simulink model "exampleModel"  (R2017b)
settings: Solver=VariableStepAuto  StartTime=0.0  StopTime=10e-6  RelTol=1e-3
PreLoadFcn:
  | setup
values from neighbouring files (symbols this model uses):
  axiClk = 156.25e6    (= 156250000)    [setup.m]    (also in setup_exampleModel_bus_axi_simulink.m; setup_exampleModel_bus_axi_simulink_lcls2.m; setup_lcls2_pcav.m)
  cav1p1_addr = 204    [setup_exampleModel_bus_axi_simulink.m]    (also in setup_exampleModel_bus_axi_simulink_lcls2.m; setup_lcls2_pcav.m; sysgen_signal.m)
  cav1p2_addr = cav1p1_addr * 2    (= 408)    [setup_exampleModel_bus_axi_simulink.m]    (also in setup_exampleModel_bus_axi_simulink_lcls2.m; setup_lcls2_pcav.m; sysgen_signal.m)
  cav2p1_addr = cav1p1_addr * 3    (= 612)    [setup_exampleModel_bus_axi_simulink.m]    (also in setup_exampleModel_bus_axi_simulink_lcls2.m; setup_lcls2_pcav.m; sysgen_signal.m)
  cav2p2_addr = cav1p1_addr * 4    (= 816)    [setup_exampleModel_bus_axi_simulink.m]    (also in setup_exampleModel_bus_axi_simulink_lcls2.m; setup_lcls2_pcav.m; sysgen_signal.m)
  Fadc = Fs/interleavedChannels    (= 29750000)    [setup.m]    (also in setup_exampleModel_bus_axi_simulink.m = 357000000; setup_exampleModel_bus_axi_simulink_lcls2.m = 351000000; setup_lcls2_pcav.m = 357000000)
  Fproc = 204e6    (= 204000000)    [setup_exampleModel_bus_axi_simulink.m]    (also in setup_exampleModel_bus_axi_simulink_lcls2.m = 200571400; setup_lcls2_pcav.m)
  Tadc = 1/fadc    (= 2.80112044818e-09)    [cavity_signal.m]    (also in setup_exampleModel_bus_axi_simulink.m; setup_exampleModel_bus_axi_simulink_lcls2.m = 2.849002849e-09; setup_lcls2_pcav.m; setup_pcav_simulink.m)
undefined symbols (not defined in the file or in its folder): AXI4, Lite
libraries: xbsIndex_r4 x248, llrf_lib x10, simulink x3
(part 2 of 3)

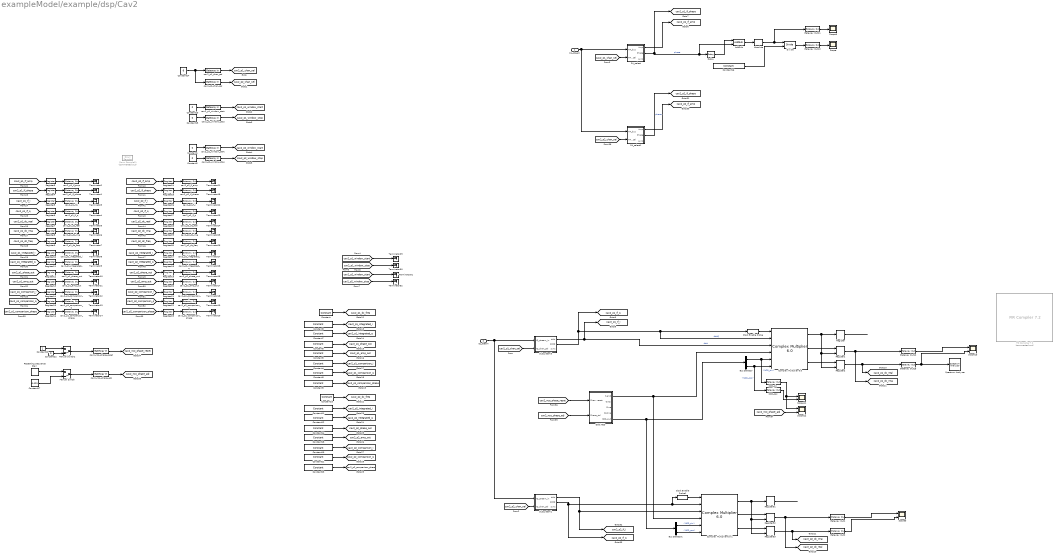
== system exampleModel/example/dsp/Cav2 ==
  PA_stream : Inport
  IQ_stream : Inport  Port=2
  Absolute : xbsIndex_r4/Absolute  precision=Full  arith_type=Unsigned  n_bits=16  bin_pt=14  quantization=Truncate  overflow=Wrap  en=off  latency=1  dbl_ovrd=off  block_type=abs
  AddSub : xbsIndex_r4/AddSub  mode=Subtraction  use_carryin=off  use_carryout=off  en=off  latency=1  precision=Full  arith_type=Unsigned  n_bits=16  bin_pt=14  quantization=Truncate  overflow=Wrap  use_behavioral_HDL=off  hw_selection=Fabric  pipelined=off  dbl_ovrd=off  block_type=addsub
  Bus Selector : BusSelector  OutputSignals=NCO_sin,NCO_cos
  Bus Selector1 : BusSelector  OutputSignals=NCO_sin,NCO_cos
  Clock Enable Probe : xbsIndex_r4/Clock Enable Probe  inherit_constraints=on  block_type=ceprobe
      settings: infoedit="Clock enable extractor.  Produces a Boolean output that mirrors the hardware clock enable associated with the input sample rate.<br><br>Hardware notes: in hardware this block costs nothing."
  Clock Enable Probe1 : xbsIndex_r4/Clock Enable Probe  inherit_constraints=on  block_type=ceprobe
      settings: infoedit="Clock enable extractor.  Produces a Boolean output that mirrors the hardware clock enable associated with the input sample rate.<br><br>Hardware notes: in hardware this block costs nothing."
  "Complex Multiplier 6.0 " : xbsIndex_r4/Complex Multiplier 6.0   hasatlast=off  hasatuser=off  atuserwidth=1  hasbtlast=off  hasbtuser=off  btuserwidth=1  multtype=Use_Mults  optimizegoal=Resources  flowcontrol=NonBlocking  outputwidth=33  roundmode=Truncate  hasctrltlast=off  hasctrltuser=off  ctrltuserwidth=1  outtlastbehv=Null  latencyconfig=Automatic  minimumlatency=15  aclken=off  aresetn=off  trim_axipin_name=on  simulation_type=hybrid_sim  simulation_model=sysgen:cmpy_v6_0  data_path_portlist={ 's_axis_a_tdata_real', 's_axis_a_tdata_imag', 's_axis_b_tdata_real', 's_axis_b_tdata_imag', 's_axis_ctrl_tdata_rounding_bit', 'm_axis_dout_tdata_real', 'm_axis_dout_tdata_imag' }  aportwidth=63  bportwidth=63  ip_name=Complex Multiplier  ip_version=6.0  dsptool_ready=true  ipcore_usecache=true  ipcore_useipmodelcache=true  ipcore_verbose=false  ipcore_latency_parameter='minimumlatency'  wrapper_available=true  port_translation_map={ 'aclken' => 'en', 'aresetn' => 'rst'}  block_type=cmpy_v6_0
  Complex Multiplier 6.0 1 : xbsIndex_r4/Complex Multiplier 6.0   hasatlast=off  hasatuser=off  atuserwidth=1  hasbtlast=off  hasbtuser=off  btuserwidth=1  multtype=Use_Mults  optimizegoal=Resources  flowcontrol=NonBlocking  outputwidth=33  roundmode=Truncate  hasctrltlast=off  hasctrltuser=off  ctrltuserwidth=1  outtlastbehv=Null  latencyconfig=Automatic  minimumlatency=15  aclken=off  aresetn=off  trim_axipin_name=on  simulation_type=hybrid_sim  simulation_model=sysgen:cmpy_v6_0  data_path_portlist={ 's_axis_a_tdata_real', 's_axis_a_tdata_imag', 's_axis_b_tdata_real', 's_axis_b_tdata_imag', 's_axis_ctrl_tdata_rounding_bit', 'm_axis_dout_tdata_real', 'm_axis_dout_tdata_imag' }  aportwidth=63  bportwidth=63  ip_name=Complex Multiplier  ip_version=6.0  dsptool_ready=true  ipcore_usecache=true  ipcore_useipmodelcache=true  ipcore_verbose=false  ipcore_latency_parameter='minimumlatency'  wrapper_available=true  port_translation_map={ 'aclken' => 'en', 'aresetn' => 'rst'}  block_type=cmpy_v6_0
  Constant : xbsIndex_r4/Constant  const=1.0  gui_display_data_type=Fixed-point  arith_type=Signed (2's comp)  n_bits=26  bin_pt=0  preci_type=Single  exp_width=8  frac_width=24  explicit_period=on  period=1/Fproc  equ=P=C  opselect=C  inp2=PCIN>>17  opr=+  inp1=P  carry=CIN  dbl_ovrd=off  block_type=constant
  Constant{1..2,13,15,22} (5 alike) : Constant  Value=0
  Constant10 : xbsIndex_r4/Constant  const=1.0  gui_display_data_type=Fixed-point  arith_type=Signed (2's comp)  n_bits=26  bin_pt=0  preci_type=Single  exp_width=8  frac_width=24  explicit_period=on  period=1/Fproc  equ=P=C  opselect=C  inp2=PCIN>>17  opr=+  inp1=P  carry=CIN  dbl_ovrd=off  block_type=constant
  Constant{3..9,11..12,14,18..19,21,23} (14 alike) : xbsIndex_r4/Constant  const=1.0  gui_display_data_type=Fixed-point  arith_type=Signed (2's comp)  n_bits=18  bin_pt=17  preci_type=Single  exp_width=8  frac_width=24  explicit_period=on  period=1/Fproc  equ=P=C  opselect=C  inp2=PCIN>>17  opr=+  inp1=P  carry=CIN  dbl_ovrd=off  block_type=constant
  Constant16 : xbsIndex_r4/Constant  const=1/(17e6)  gui_display_data_type=Fixed-point  arith_type=Signed (2's comp)  n_bits=32  bin_pt=31  preci_type=Single  exp_width=8  frac_width=24  explicit_period=on  period=1  equ=P=C  opselect=C  inp2=PCIN>>17  opr=+  inp1=P  carry=CIN  dbl_ovrd=off  block_type=constant
  Constant17 : Constant  Value=0.023
  Constant20 : Constant
  Constant24 : Constant  Value=6
  DDC NCO : Subsystem
  Delay : xbsIndex_r4/Delay  rst=off  infoeditControl=Selection of Reset will increase slice count due to use of real FFs and instead of SRLs  en=off  latency=1  reg_retiming=off  dbl_ovrd=off  block_type=delay
  Divide : xbsIndex_r4/Divide  flow_control=NonBlocking  axi_optimize_goal=Resources  algorithm_type=Radix2  infoedit1=Specify output fraction-width for Fixed-point division.  fractional_width=12  infoedit2=Specify latency for Floating-point division.  latency=1  rate=1  has_a_tlast=off  has_a_tuser=off  has_b_tlast=off  has_b_tuser=off  en=off  has_result_tready=off  result_tlast_behv=Pass_A_TLAST  has_underflow=off  has_overflow=off  has_invalid_op=off  has_divide_by_zero=off  fpo_op_type=mergeddivide  block_type=divide
      settings: infoedit=Blocking: Wait for data on all inputs, allow back-pressure.<br>NonBlocking: operate every cycle in which all inputs are valid, no back-pressure.
  Down Sample11 : xbsIndex_r4/Down Sample  Commented=on  sample_ratio=8  sample_phase="Last Value of Frame  (most efficient)"  en=off  rst=off  latency=1  dbl_ovrd=off  block_type=dsamp
  "FIR Compiler 7.2 " : xbsIndex_r4/FIR Compiler 7.2   Commented=on  coefficientvector=[6,0,-4,-3,5,6,-6,-13,7,44,64,44,7,-13,-6,6,5,-3,-4,0,6]  coefficient_sets=1  coefficient_reload=off  filter_type=Single_Rate  rate_change_type=Integer  interpolation_rate=1  decimation_rate=1  zero_pack_factor=1  channel_sequence=Basic  number_channels=1  pattern_list='P4-0,P4-1,P4-2,P4-3,P4-4'  number_paths=1  ratespecification=Maximum_Possible  sampleperiod=1  hardwareoversamplingrate=1  coefficient_sign=Signed  quantization=Integer_Coefficients  coefficient_width=16  bestprecision=on  coefficient_fractional_bits=0  coefficient_structure=Inferred  output_rounding_mode=Full_Precision  output_width=24  filter_architecture=Systolic_Multiply_Accumulate  optimization_goal=Area  optimization_list='None'  data_buffer_type=Automatic  coefficient_buffer_type=Automatic  input_buffer_type=Automatic  output_buffer_type=Automatic  preference_for_other_storage=Automatic  multi_column_support=Automatic  columnconfig='1'  inter_column_pipe_length=4  data_has_tlast=Not_Required  m_data_has_tready=off  s_data_has_fifo=off  s_data_has_tuser=Not_Required  m_data_has_tuser=Not_Required  s_config_sync_mode=On_Vector  s_config_method=Single  num_reload_slots=1  has_aclken=off  has_aresetn=off  infoeditControl=ARESETn must be asserted for a minimum of 2 cycles  reset_data_vector=on  trim_axipin_name=on  simulation_type=hybrid_sim  simulation_model=sysgen:xfirv7_2_cmodel  data_path_portlist={ 's_axis_data_tdata', 'm_axis_data_tdata' }  passband_min=0.0  passband_max=0.5  stopband_min=0.5  stopband_max=1.0  filter_selection=1  gui_behaviour=Sysgen_GUI  data_sign=Signed  data_width=16  data_fractional_bits=0  data_tuser_width=1  wrapper_available=true  ip_wrap_arbitrary_binary_point=true  ip_name=FIR Compiler  ip_version=7.2  dsptool_ready=true  ipcore_usecache=true  ipcore_useipmodelcache=true  port_translation_map={ 'aclken' => 'en', 'aresetn' => 'rst' }  run_core_at_system_period=true  ipcore_xco_need_fpga_part=true  block_type=fir_compiler_v7_2
      settings: infoedit=Maximum Possible : Maximizes oversampling rate. Abstracted input handshake (no s_data_tvalid) and automatic rate propagation.<br>Hardware Oversampling Rate : Specifies oversampling rate relative to the input sample period. Abstracted input handshake (no s_data_tvalid) and automatic rate propagation.<br>Input/Output Sample Period : Specifies absolute oversampling rate. No input handshake abstraction (exposes s_data_tvalid) and no rate propagation.
  Gateway Out{1..2,10..12,15} (6 alike) : xbsIndex_r4/Gateway Out  inherit_from_input=off  hdl_port=off  rows=1  columns=1  UseAsDAC=off  DACChannel='1'  interface=None  automatic_assignment=on  address_offset=hex2dec('00')  intf_name=''  intf_description=''  timing_constraint=None  locs_specified=off  LOCs={}  io_standard={}  block_type=gatewayout
  Manual Switch : ManualSwitch  CurrentSetting=0
  Manual Switch2 : ManualSwitch  CurrentSetting=0
  NCO_cos : xbsIndex_r4/Gateway Out  inherit_from_input=off  hdl_port=off  rows=1  columns=1  UseAsDAC=off  DACChannel='1'  interface=None  automatic_assignment=on  address_offset=hex2dec('00')  intf_name=''  intf_description=''  timing_constraint=None  locs_specified=off  LOCs={}  io_standard={}  block_type=gatewayout
  NCO_sin : xbsIndex_r4/Gateway Out  inherit_from_input=off  hdl_port=off  rows=1  columns=1  UseAsDAC=off  DACChannel='1'  interface=None  automatic_assignment=on  address_offset=hex2dec('00')  intf_name=''  intf_description=''  timing_constraint=None  locs_specified=off  LOCs={}  io_standard={}  block_type=gatewayout
  PA_select : Subsystem
  PA_select1 : Subsystem
  Register{,3..31} (30 alike) : xbsIndex_r4/Register  init=0  rst=off  en=off  dbl_ovrd=off  block_type=register
  Register{1..2,32..33} (4 alike) : xbsIndex_r4/Register  init=0  rst=off  en=on  dbl_ovrd=off  block_type=register
  Repeating Sequence Stair : simulink/Sources/Repeating Sequence Stair  OutValues=[0 (30/360) (45/360) (60/360) (75/360) (90/360) (8.2941/360)]  tsamp=0.5e-6  OutMin=[]  OutMax=[]  OutDataTypeStr=double  OutputDataTypeScalingMode=double  OutDataType=fixdt(0,8)  ConRadixGroup=Best Precision: Vector-wise  OutScaling=2^-12
  Scope : Scope
  Scope{3,11..13} (4 alike) : Scope  NumInputPorts=2
  Scope9 : Scope
  Spectrum Analyzer : SpectrumAnalyzer
  Subsystem1 : Subsystem
  Subsystem3 : Subsystem
  Terminator{1..32} (32 alike) : Terminator
  cav1_p1_comparison_q : xbsIndex_r4/Gateway Out  inherit_from_input=off  hdl_port=on  rows=1  columns=1  UseAsDAC=off  DACChannel='1'  interface=AXI4-Lite  automatic_assignment=off  address_offset=cav2p1_addr+hex2dec('3c')  intf_name='cav2_p1_comparison_q'  intf_description=''  timing_constraint=None  locs_specified=off  LOCs={}  io_standard={}  block_type=gatewayout
  cav2_nco_phase_adj : xbsIndex_r4/Gateway In  gui_display_data_type=Fixed-point  arith_type=Unsigned  n_bits=29  bin_pt=29  preci_type=Single  exp_width=8  frac_width=24  rows=1  columns=1  quantization="Round  (unbiased: +/- Inf)"  overflow=Saturate  period=1/Fproc  UseAsADC=off  ADCChannel='1'  interface=AXI4-Lite  automatic_assignment=off  address_offset=cav2p1_addr+hex2dec('4c')  intf_name='cav1_nco_phase_adj'  intf_description=''  default_value=0  timing_constraint=None  locs_specified=off  LOCs={}  io_standard={}  inherit_from_input=off  hdl_port=on  dbl_ovrd=off  block_type=gatewayin
  cav2_nco_phase_reset : xbsIndex_r4/Gateway In  gui_display_data_type=Fixed-point  arith_type=Unsigned  n_bits=1  bin_pt=0  preci_type=Single  exp_width=8  frac_width=24  rows=1  columns=1  quantization="Round  (unbiased: +/- Inf)"  overflow=Saturate  period=1/Fproc  UseAsADC=off  ADCChannel='1'  interface=AXI4-Lite  automatic_assignment=off  address_offset=cav2p1_addr+hex2dec('50')  intf_name='cav1_nco_phase_reset'  intf_description=''  default_value=0  timing_constraint=None  locs_specified=off  LOCs={}  io_standard={}  inherit_from_input=off  hdl_port=on  dbl_ovrd=off  block_type=gatewayin
  cav2_p1_amp_out : xbsIndex_r4/Gateway Out  inherit_from_input=off  hdl_port=on  rows=1  columns=1  UseAsDAC=off  DACChannel='1'  interface=AXI4-Lite  automatic_assignment=off  address_offset=cav2p1_addr+hex2dec('34')  intf_name='cav2_p1_amp_out'  intf_description=''  timing_constraint=None  locs_specified=off  LOCs={}  io_standard={}  block_type=gatewayout
  cav2_p1_chan_sel : xbsIndex_r4/Gateway In  gui_display_data_type=Fixed-point  arith_type=Unsigned  n_bits=4  bin_pt=0  preci_type=Single  exp_width=8  frac_width=24  rows=1  columns=1  quantization="Round  (unbiased: +/- Inf)"  overflow=Saturate  period=1/Fproc  UseAsADC=off  ADCChannel='1'  interface=AXI4-Lite  automatic_assignment=off  address_offset=cav2p1_addr+hex2dec('10')  intf_name='cav2_p1_chan_sel'  intf_description=''  default_value=0  timing_constraint=None  locs_specified=off  LOCs={}  io_standard={}  inherit_from_input=off  hdl_port=on  dbl_ovrd=off  block_type=gatewayin
  cav2_p1_comparison_i : xbsIndex_r4/Gateway Out  inherit_from_input=off  hdl_port=on  rows=1  columns=1  UseAsDAC=off  DACChannel='1'  interface=AXI4-Lite  automatic_assignment=off  address_offset=cav2p1_addr+hex2dec('38')  intf_name='cav2_p1_comparison_i'  intf_description=''  timing_constraint=None  locs_specified=off  LOCs={}  io_standard={}  block_type=gatewayout
  cav2_p1_comparison_phase : xbsIndex_r4/Gateway Out  inherit_from_input=off  hdl_port=on  rows=1  columns=1  UseAsDAC=off  DACChannel='1'  interface=AXI4-Lite  automatic_assignment=off  address_offset=cav2p1_addr+hex2dec('40')  intf_name='cav2_p1_comparison_phase'  intf_description=''  timing_constraint=None  locs_specified=off  LOCs={}  io_standard={}  block_type=gatewayout
  cav2_p1_dc_freq : xbsIndex_r4/Gateway Out  inherit_from_input=off  hdl_port=on  rows=1  columns=1  UseAsDAC=off  DACChannel='1'  interface=AXI4-Lite  automatic_assignment=off  address_offset=cav2p1_addr+hex2dec('24')  intf_name='cav2_p1_dc_freq'  intf_description=''  timing_constraint=None  locs_specified=off  LOCs={}  io_standard={}  block_type=gatewayout
  cav2_p1_dc_img : xbsIndex_r4/Gateway Out  inherit_from_input=off  hdl_port=on  rows=1  columns=1  UseAsDAC=off  DACChannel='1'  interface=AXI4-Lite  automatic_assignment=off  address_offset=cav2p1_addr+hex2dec('18')  intf_name='cav2_p1_dc_img'  intf_description=''  timing_constraint=None  locs_specified=off  LOCs={}  io_standard={}  block_type=gatewayout
  cav2_p1_dc_real : xbsIndex_r4/Gateway Out  inherit_from_input=off  hdl_port=on  rows=1  columns=1  UseAsDAC=off  DACChannel='1'  interface=AXI4-Lite  automatic_assignment=off  address_offset=cav2p1_addr+hex2dec('14')  intf_name='cav2_p1_dc_real'  intf_description=''  timing_constraint=None  locs_specified=off  LOCs={}  io_standard={}  block_type=gatewayout
  cav2_p1_if_amp : xbsIndex_r4/Gateway Out  inherit_from_input=off  hdl_port=on  rows=1  columns=1  UseAsDAC=off  DACChannel='1'  interface=AXI4-Lite  automatic_assignment=off  address_offset=cav2p1_addr+hex2dec('0')  intf_name='cav2_p1_if_amp'  intf_description=''  timing_constraint=None  locs_specified=off  LOCs={}  io_standard={}  block_type=gatewayout
  cav2_p1_if_i : xbsIndex_r4/Gateway Out  inherit_from_input=off  hdl_port=on  rows=1  columns=1  UseAsDAC=off  DACChannel='1'  interface=AXI4-Lite  automatic_assignment=off  address_offset=cav2p1_addr+hex2dec('8')  intf_name='cav2_p1_if_i'  intf_description=''  timing_constraint=None  locs_specified=off  LOCs={}  io_standard={}  block_type=gatewayout
  cav2_p1_if_phase : xbsIndex_r4/Gateway Out  inherit_from_input=off  hdl_port=on  rows=1  columns=1  UseAsDAC=off  DACChannel='1'  interface=AXI4-Lite  automatic_assignment=off  address_offset=cav2p1_addr+hex2dec('4')  intf_name='cav2_p1_if_phase'  intf_description=''  timing_constraint=None  locs_specified=off  LOCs={}  io_standard={}  block_type=gatewayout
  cav2_p1_if_q : xbsIndex_r4/Gateway Out  inherit_from_input=off  hdl_port=on  rows=1  columns=1  UseAsDAC=off  DACChannel='1'  interface=AXI4-Lite  automatic_assignment=off  address_offset=cav2p1_addr+hex2dec('c')  intf_name='cav2_p1_if_q'  intf_description=''  timing_constraint=None  locs_specified=off  LOCs={}  io_standard={}  block_type=gatewayout
  cav2_p1_integrated_i : xbsIndex_r4/Gateway Out  inherit_from_input=off  hdl_port=on  rows=1  columns=1  UseAsDAC=off  DACChannel='1'  interface=AXI4-Lite  automatic_assignment=off  address_offset=cav2p1_addr+hex2dec('28')  intf_name='cav2_p1_integrated_i'  intf_description=''  timing_constraint=None  locs_specified=off  LOCs={}  io_standard={}  block_type=gatewayout
  cav2_p1_integrated_q : xbsIndex_r4/Gateway Out  inherit_from_input=off  hdl_port=on  rows=1  columns=1  UseAsDAC=off  DACChannel='1'  interface=AXI4-Lite  automatic_assignment=off  address_offset=cav2p1_addr+hex2dec('2c')  intf_name='cav2_p1_integrated_q'  intf_description=''  timing_constraint=None  locs_specified=off  LOCs={}  io_standard={}  block_type=gatewayout
  cav2_p1_phase_out : xbsIndex_r4/Gateway Out  inherit_from_input=off  hdl_port=on  rows=1  columns=1  UseAsDAC=off  DACChannel='1'  interface=AXI4-Lite  automatic_assignment=off  address_offset=cav2p1_addr+hex2dec('30')  intf_name='cav2_p1_phase_out'  intf_description=''  timing_constraint=None  locs_specified=off  LOCs={}  io_standard={}  block_type=gatewayout
  cav2_p1_window_start : xbsIndex_r4/Gateway In  gui_display_data_type=Fixed-point  arith_type=Unsigned  n_bits=16  bin_pt=0  preci_type=Single  exp_width=8  frac_width=24  rows=1  columns=1  quantization="Round  (unbiased: +/- Inf)"  overflow=Saturate  period=1/Fproc  UseAsADC=off  ADCChannel='1'  interface=AXI4-Lite  automatic_assignment=off  address_offset=cav2p1_addr+hex2dec('1c')  intf_name='cav2_p1_window_start'  intf_description=''  default_value=0  timing_constraint=None  locs_specified=off  LOCs={}  io_standard={}  inherit_from_input=off  hdl_port=on  dbl_ovrd=off  block_type=gatewayin
  cav2_p1_window_stop : xbsIndex_r4/Gateway In  gui_display_data_type=Fixed-point  arith_type=Unsigned  n_bits=16  bin_pt=0  preci_type=Single  exp_width=8  frac_width=24  rows=1  columns=1  quantization="Round  (unbiased: +/- Inf)"  overflow=Saturate  period=1/Fproc  UseAsADC=off  ADCChannel='1'  interface=AXI4-Lite  automatic_assignment=off  address_offset=cav2p1_addr+hex2dec('20')  intf_name='cav2_p1_window_stop'  intf_description=''  default_value=0  timing_constraint=None  locs_specified=off  LOCs={}  io_standard={}  inherit_from_input=off  hdl_port=on  dbl_ovrd=off  block_type=gatewayin
  cav2_p2_amp_out : xbsIndex_r4/Gateway Out  inherit_from_input=off  hdl_port=on  rows=1  columns=1  UseAsDAC=off  DACChannel='1'  interface=AXI4-Lite  automatic_assignment=off  address_offset=cav2p2_addr+hex2dec('34')  intf_name='cav2_p2_amp_out'  intf_description=''  timing_constraint=None  locs_specified=off  LOCs={}  io_standard={}  block_type=gatewayout
  cav2_p2_chan_sel : xbsIndex_r4/Gateway In  gui_display_data_type=Fixed-point  arith_type=Unsigned  n_bits=4  bin_pt=0  preci_type=Single  exp_width=8  frac_width=24  rows=1  columns=1  quantization="Round  (unbiased: +/- Inf)"  overflow=Saturate  period=1/Fproc  UseAsADC=off  ADCChannel='1'  interface=AXI4-Lite  automatic_assignment=off  address_offset=cav2p2_addr+hex2dec('10')  intf_name='cav2_p2_chan_sel'  intf_description=''  default_value=0  timing_constraint=None  locs_specified=off  LOCs={}  io_standard={}  inherit_from_input=off  hdl_port=on  dbl_ovrd=off  block_type=gatewayin
  cav2_p2_comparison_i : xbsIndex_r4/Gateway Out  inherit_from_input=off  hdl_port=on  rows=1  columns=1  UseAsDAC=off  DACChannel='1'  interface=AXI4-Lite  automatic_assignment=off  address_offset=cav2p2_addr+hex2dec('38')  intf_name='cav2_p2_comparison_i'  intf_description=''  timing_constraint=None  locs_specified=off  LOCs={}  io_standard={}  block_type=gatewayout
  cav2_p2_comparison_phase : xbsIndex_r4/Gateway Out  inherit_from_input=off  hdl_port=on  rows=1  columns=1  UseAsDAC=off  DACChannel='1'  interface=AXI4-Lite  automatic_assignment=off  address_offset=cav2p2_addr+hex2dec('40')  intf_name='cav2_p2_comparison_phase'  intf_description=''  timing_constraint=None  locs_specified=off  LOCs={}  io_standard={}  block_type=gatewayout
  cav2_p2_comparison_q : xbsIndex_r4/Gateway Out  inherit_from_input=off  hdl_port=on  rows=1  columns=1  UseAsDAC=off  DACChannel='1'  interface=AXI4-Lite  automatic_assignment=off  address_offset=cav2p2_addr+hex2dec('3c')  intf_name='cav2_p2_comparison_q'  intf_description=''  timing_constraint=None  locs_specified=off  LOCs={}  io_standard={}  block_type=gatewayout
  cav2_p2_dc_freq : xbsIndex_r4/Gateway Out  inherit_from_input=off  hdl_port=on  rows=1  columns=1  UseAsDAC=off  DACChannel='1'  interface=AXI4-Lite  automatic_assignment=off  address_offset=cav2p2_addr+hex2dec('24')  intf_name='cav2_p2_dc_freq'  intf_description=''  timing_constraint=None  locs_specified=off  LOCs={}  io_standard={}  block_type=gatewayout
  cav2_p2_dc_img : xbsIndex_r4/Gateway Out  inherit_from_input=off  hdl_port=on  rows=1  columns=1  UseAsDAC=off  DACChannel='1'  interface=AXI4-Lite  automatic_assignment=off  address_offset=cav2p2_addr+hex2dec('18')  intf_name='cav2_p2_dc_img'  intf_description=''  timing_constraint=None  locs_specified=off  LOCs={}  io_standard={}  block_type=gatewayout
  cav2_p2_dc_real : xbsIndex_r4/Gateway Out  inherit_from_input=off  hdl_port=on  rows=1  columns=1  UseAsDAC=off  DACChannel='1'  interface=AXI4-Lite  automatic_assignment=off  address_offset=cav2p2_addr+hex2dec('14')  intf_name='cav2_p2_dc_real'  intf_description=''  timing_constraint=None  locs_specified=off  LOCs={}  io_standard={}  block_type=gatewayout
  cav2_p2_if_amp : xbsIndex_r4/Gateway Out  inherit_from_input=off  hdl_port=on  rows=1  columns=1  UseAsDAC=off  DACChannel='1'  interface=AXI4-Lite  automatic_assignment=off  address_offset=cav2p2_addr+hex2dec('0')  intf_name='cav2_p2_if_amp'  intf_description=''  timing_constraint=None  locs_specified=off  LOCs={}  io_standard={}  block_type=gatewayout
  "cav2_p2_if_i " : xbsIndex_r4/Gateway Out  inherit_from_input=off  hdl_port=on  rows=1  columns=1  UseAsDAC=off  DACChannel='1'  interface=AXI4-Lite  automatic_assignment=off  address_offset=cav2p2_addr+hex2dec('8')  intf_name='cav2_p2_if_i'  intf_description=''  timing_constraint=None  locs_specified=off  LOCs={}  io_standard={}  block_type=gatewayout
  cav2_p2_if_phase : xbsIndex_r4/Gateway Out  inherit_from_input=off  hdl_port=on  rows=1  columns=1  UseAsDAC=off  DACChannel='1'  interface=AXI4-Lite  automatic_assignment=off  address_offset=cav2p2_addr+hex2dec('4')  intf_name='cav2_p2_if_phase'  intf_description=''  timing_constraint=None  locs_specified=off  LOCs={}  io_standard={}  block_type=gatewayout
  cav2_p2_if_q : xbsIndex_r4/Gateway Out  inherit_from_input=off  hdl_port=on  rows=1  columns=1  UseAsDAC=off  DACChannel='1'  interface=AXI4-Lite  automatic_assignment=off  address_offset=cav2p2_addr+hex2dec('c')  intf_name='cav2_p2_if_q'  intf_description=''  timing_constraint=None  locs_specified=off  LOCs={}  io_standard={}  block_type=gatewayout
  cav2_p2_integrated_i : xbsIndex_r4/Gateway Out  inherit_from_input=off  hdl_port=on  rows=1  columns=1  UseAsDAC=off  DACChannel='1'  interface=AXI4-Lite  automatic_assignment=off  address_offset=cav2p2_addr+hex2dec('28')  intf_name='cav2_p2_integrated_i'  intf_description=''  timing_constraint=None  locs_specified=off  LOCs={}  io_standard={}  block_type=gatewayout
  cav2_p2_integrated_q : xbsIndex_r4/Gateway Out  inherit_from_input=off  hdl_port=on  rows=1  columns=1  UseAsDAC=off  DACChannel='1'  interface=AXI4-Lite  automatic_assignment=off  address_offset=cav2p2_addr+hex2dec('2c')  intf_name='cav2_p2_integrated_q'  intf_description=''  timing_constraint=None  locs_specified=off  LOCs={}  io_standard={}  block_type=gatewayout
  cav2_p2_phase_out : xbsIndex_r4/Gateway Out  inherit_from_input=off  hdl_port=on  rows=1  columns=1  UseAsDAC=off  DACChannel='1'  interface=AXI4-Lite  automatic_assignment=off  address_offset=cav2p2_addr+hex2dec('30')  intf_name='cav2_p2_phase_out'  intf_description=''  timing_constraint=None  locs_specified=off  LOCs={}  io_standard={}  block_type=gatewayout
  cav2_p2_window_start : xbsIndex_r4/Gateway In  gui_display_data_type=Fixed-point  arith_type=Unsigned  n_bits=16  bin_pt=0  preci_type=Single  exp_width=8  frac_width=24  rows=1  columns=1  quantization="Round  (unbiased: +/- Inf)"  overflow=Saturate  period=1/Fproc  UseAsADC=off  ADCChannel='1'  interface=AXI4-Lite  automatic_assignment=off  address_offset=cav2p2_addr+hex2dec('1c')  intf_name='cav2_p2_window_start'  intf_description=''  default_value=0  timing_constraint=None  locs_specified=off  LOCs={}  io_standard={}  inherit_from_input=off  hdl_port=on  dbl_ovrd=off  block_type=gatewayin
  cav2_p2_window_stop : xbsIndex_r4/Gateway In  gui_display_data_type=Fixed-point  arith_type=Unsigned  n_bits=16  bin_pt=0  preci_type=Single  exp_width=8  frac_width=24  rows=1  columns=1  quantization="Round  (unbiased: +/- Inf)"  overflow=Saturate  period=1/Fproc  UseAsADC=off  ADCChannel='1'  interface=AXI4-Lite  automatic_assignment=off  address_offset=cav2p2_addr+hex2dec('20')  intf_name='cav2_p2_window_stop'  intf_description=''  default_value=0  timing_constraint=None  locs_specified=off  LOCs={}  io_standard={}  inherit_from_input=off  hdl_port=on  dbl_ovrd=off  block_type=gatewayin
  tag scope: cav2_nco_phase_adj=global, cav2_nco_phase_reset=global, cav2_p1_amp_out=global, cav2_p1_chan_sel=global, cav2_p1_comparison_i=global, cav2_p1_comparison_phase=global, cav2_p1_comparison_q=global, cav2_p1_dc_freq=global, cav2_p1_dc_img=global, cav2_p1_dc_real=global, cav2_p1_if_amp=global, cav2_p1_if_i=global, cav2_p1_if_phase=global, cav2_p1_if_q=global, cav2_p1_integrated_i=global, cav2_p1_integrated_q=global, cav2_p1_phase_out=global, cav2_p1_window_start=global, cav2_p1_window_stop=global, cav2_p2_amp_out=global, cav2_p2_chan_sel=global, cav2_p2_comparison_i=global, cav2_p2_comparison_phase=global, cav2_p2_comparison_q=global, cav2_p2_dc_freq=global, cav2_p2_dc_img=global, cav2_p2_dc_real=global, cav2_p2_if_amp=global, cav2_p2_if_i=global, cav2_p2_if_phase=global, cav2_p2_if_q=global, cav2_p2_integrated_i=global, cav2_p2_integrated_q=global, cav2_p2_phase_out=global, cav2_p2_window_start=global, cav2_p2_window_stop=global
  wires:
  Constant24/1 -> cav2_p1_chan_sel/1, cav2_p2_chan_sel/1
  Constant10/1 -> [cav2_p2_dc_freq]
  Constant11/1 -> [cav2_p2_integrated_i]
  Constant12/1 -> [cav2_p2_integrated_q]
  Constant14/1 -> [cav2_p2_phase_out]
  Constant18/1 -> [cav2_p2_amp_out]
  Constant19/1 -> [cav2_p2_comparison_i]
  Constant21/1 -> [cav2_p2_comparison_q]
  Constant23/1 -> [cav2_p2_comparison_phase]
  Constant9/1 -> [cav2_p1_comparison_phase]
  Constant3/1 -> [cav2_p1_comparison_q]
  Constant4/1 -> [cav2_p1_comparison_i]
  Constant5/1 -> [cav2_p1_amp_out]
  Constant6/1 -> [cav2_p1_phase_out]
  Constant7/1 -> [cav2_p1_integrated_q]
  Constant8/1 -> [cav2_p1_integrated_i]
  Constant/1 -> [cav2_p1_dc_freq]
  [cav2_p2_window_start] -> Terminator31/1
  [cav2_p2_window_stop] -> Terminator32/1
  [cav2_p1_window_stop] -> Terminator30/1
  [cav2_p1_window_start] -> Terminator29/1
  Subsystem1/2(ddcQ) -> [cav2_p2_if_q], Complex Multiplier 6.0 1/2, Clock Enable Probe1/1
  Subsystem1/1(ddcI) -> [cav2_p2_if_i], Complex Multiplier 6.0 1/3
  Complex Multiplier 6.0 1/3 -> Register33/1
  Gateway Out1/1 -> Scope3/1
  Register33/1 -> Gateway Out2/1, [cav2_p2_dc_img]
  Bus Selector1/1 -> Complex Multiplier 6.0 1/5  "<NCO_sin>"
  Gateway Out2/1 -> Scope3/2
  Bus Selector1/2 -> Complex Multiplier 6.0 1/6  "<NCO_cos>"
  Complex Multiplier 6.0 1/1 -> Register31/1, Register32/2, Register33/2
  Register31/1 -> ?
  Clock Enable Probe1/1 -> Complex Multiplier 6.0 1/1
  Register32/1 -> Gateway Out1/1, [cav2_p2_dc_real]
  Complex Multiplier 6.0 1/2 -> Register32/1
  [cav2_p2_chan_sel] -> Subsystem1/2(IQ_chan_sel)
  Register23/1 -> cav2_p2_comparison_phase/1
  Register22/1 -> cav2_p2_comparison_q/1
  Register21/1 -> cav2_p2_comparison_i/1
  Register20/1 -> cav2_p2_amp_out/1
  Register19/1 -> cav2_p2_phase_out/1
  Register18/1 -> cav2_p2_integrated_q/1
  Register17/1 -> cav2_p2_integrated_i/1
  Register30/1 -> cav2_p2_dc_freq/1
  Register29/1 -> cav2_p2_dc_img/1
  Register28/1 -> cav2_p2_dc_real/1
  Register27/1 -> cav2_p2_if_q/1
  Register26/1 -> "cav2_p2_if_i "/1
  Register25/1 -> cav2_p2_if_phase/1
  Register24/1 -> cav2_p2_if_amp/1
  [cav2_p2_if_amp] -> Register24/1
  [cav2_p2_comparison_phase] -> Register23/1
  [cav2_p2_comparison_q] -> Register22/1
  [cav2_p2_comparison_i] -> Register21/1
  [cav2_p2_amp_out] -> Register20/1
  [cav2_p2_phase_out] -> Register19/1
  [cav2_p2_integrated_q] -> Register18/1
  [cav2_p2_integrated_i] -> Register17/1
  [cav2_p2_dc_freq] -> Register30/1
  [cav2_p2_dc_img] -> Register29/1
  [cav2_p2_dc_real] -> Register28/1
  [cav2_p2_if_q] -> Register27/1
  [cav2_p2_if_i] -> Register26/1
  [cav2_p2_if_phase] -> Register25/1
  cav2_p2_if_phase/1 -> Terminator15/1
  "cav2_p2_if_i "/1 -> Terminator22/1
  cav2_p2_if_amp/1 -> Terminator21/1
  cav2_p2_if_q/1 -> Terminator23/1
  cav2_p2_dc_real/1 -> Terminator24/1
  cav2_p2_dc_img/1 -> Terminator25/1
  cav2_p2_dc_freq/1 -> Terminator26/1
  cav2_p2_integrated_i/1 -> Terminator27/1
  cav2_p2_integrated_q/1 -> Terminator28/1
  cav2_p2_phase_out/1 -> Terminator16/1
  cav2_p2_amp_out/1 -> Terminator17/1
  cav2_p2_comparison_i/1 -> Terminator18/1
  cav2_p2_comparison_q/1 -> Terminator19/1
  cav2_p2_comparison_phase/1 -> Terminator20/1
  PA_stream/1 -> PA_select/1(PA_bus), PA_select1/1(PA_bus)
  PA_select1/1(Amp) -> [cav2_p2_if_amp]
  PA_select1/2(Phase) -> [cav2_p2_if_phase]  "phase"
  [cav2_p2_chan_sel] -> PA_select1/2(PA_chan_sel)
  cav2_nco_phase_adj/1 -> [cav2_nco_phase_adj]
  [cav2_nco_phase_adj] -> Scope12/2
  Repeating Sequence Stair/1 -> Manual Switch/1
  Constant17/1 -> Manual Switch/2
  Manual Switch/1 -> cav2_nco_phase_adj/1
  cav2_nco_phase_reset/1 -> [cav2_nco_phase_reset]
  Manual Switch2/1 -> cav2_nco_phase_reset/1
  Constant20/1 -> Manual Switch2/1
  Constant22/1 -> Manual Switch2/2
  cav2_p1_comparison_phase/1 -> Terminator14/1
  cav1_p1_comparison_q/1 -> Terminator13/1
  cav2_p1_comparison_i/1 -> Terminator12/1
  cav2_p1_amp_out/1 -> Terminator11/1
  cav2_p1_phase_out/1 -> Terminator10/1
  cav2_p1_integrated_q/1 -> Terminator9/1
  cav2_p1_integrated_i/1 -> Terminator8/1
  cav2_p1_dc_freq/1 -> Terminator7/1
  cav2_p1_dc_img/1 -> Terminator6/1
  cav2_p1_dc_real/1 -> Terminator5/1
  cav2_p1_if_q/1 -> Terminator4/1
  [cav2_p1_if_phase] -> Register4/1
  [cav2_p1_if_i] -> Register5/1
  [cav2_p1_if_q] -> Register6/1
  [cav2_p1_dc_real] -> Register7/1
  [cav2_p1_dc_img] -> Register8/1
  [cav2_p1_dc_freq] -> Register9/1
  [cav2_p1_integrated_i] -> Register10/1
  [cav2_p1_integrated_q] -> Register11/1
  [cav2_p1_phase_out] -> Register12/1
  [cav2_p1_amp_out] -> Register13/1
  [cav2_p1_comparison_i] -> Register14/1
  [cav2_p1_comparison_q] -> Register15/1
  [cav2_p1_comparison_phase] -> Register16/1
  Register14/1 -> cav2_p1_comparison_i/1
  Register13/1 -> cav2_p1_amp_out/1
  Register12/1 -> cav2_p1_phase_out/1
  Register11/1 -> cav2_p1_integrated_q/1
  Register10/1 -> cav2_p1_integrated_i/1
  Register9/1 -> cav2_p1_dc_freq/1
  Register8/1 -> cav2_p1_dc_img/1
  Register7/1 -> cav2_p1_dc_real/1
  Register6/1 -> cav2_p1_if_q/1
  Register5/1 -> cav2_p1_if_i/1
  Register4/1 -> cav2_p1_if_phase/1
  Register15/1 -> cav1_p1_comparison_q/1
  Register16/1 -> cav2_p1_comparison_phase/1
  cav2_p1_if_amp/1 -> Terminator2/1
  Register3/1 -> cav2_p1_if_amp/1
  [cav2_p1_if_amp] -> Register3/1
  cav2_p1_if_i/1 -> Terminator3/1
  cav2_p1_if_phase/1 -> Terminator1/1
  cav2_p2_chan_sel/1 -> [cav2_p2_chan_sel]
  cav2_p1_chan_sel/1 -> [cav2_p1_chan_sel]
  [cav2_p1_chan_sel] -> Subsystem3/2(IQ_chan_sel)
  [cav2_p1_chan_sel] -> PA_select/2(PA_chan_sel)
  cav2_p2_window_start/1 -> [cav2_p2_window_start]
  Constant2/1 -> cav2_p2_window_stop/1
  Constant1/1 -> cav2_p2_window_start/1
  cav2_p2_window_stop/1 -> [cav2_p2_window_stop]
  Constant13/1 -> cav2_p1_window_start/1
  cav2_p1_window_stop/1 -> [cav2_p1_window_stop]
  cav2_p1_window_start/1 -> [cav2_p1_window_start]
  Constant15/1 -> cav2_p1_window_stop/1
  IQ_stream/1 -> Subsystem3/1(IQ_stream_in), Subsystem1/1(IQ_stream_in)
  Gateway Out15/1 -> Spectrum Analyzer/1, Scope13/2
  Gateway Out12/1 -> Scope13/1
  Clock Enable Probe/1 -> "Complex Multiplier 6.0 "/1
  NCO_sin/1 -> Scope11/1, Scope12/1
  NCO_cos/1 -> Scope11/2
  Absolute/1 -> Divide/1, Gateway Out11/1
  Gateway Out11/1 -> Scope9/1
  Gateway Out10/1 -> Scope/1
  Divide/1 -> Gateway Out10/1
  Constant16/1 -> Divide/2
  Delay/1 -> AddSub/1
  AddSub/1 -> Absolute/1
  Subsystem3/1(ddcI) -> "Complex Multiplier 6.0 "/3, [cav2_p1_if_i]  "ddcI"
  Subsystem3/2(ddcQ) -> Clock Enable Probe/1, "Complex Multiplier 6.0 "/2, [cav2_p1_if_q]  "ddcQ"
  PA_select/2(Phase) -> Delay/1, AddSub/2, [cav2_p1_if_phase]  "phase"
  Register/1 -> ?
  DDC NCO/5(NCO_out) -> Bus Selector/1, Bus Selector1/1
  Register2/1 -> Gateway Out15/1, [cav2_p1_dc_real]
  Bus Selector/1 -> "Complex Multiplier 6.0 "/5, NCO_sin/1  "<NCO_sin>"
  [cav2_nco_phase_reset] -> DDC NCO/1(Phase_reset)
  Register1/1 -> Gateway Out12/1, [cav2_p1_dc_img]
  [cav2_nco_phase_adj] -> DDC NCO/2(Phase_ctrl)
  DDC NCO/1(tvalid) -> "Complex Multiplier 6.0 "/4, Complex Multiplier 6.0 1/4
  "Complex Multiplier 6.0 "/1 -> Register/1, Register1/2, Register2/2
  "Complex Multiplier 6.0 "/3 -> Register2/1
  Bus Selector/2 -> "Complex Multiplier 6.0 "/6, NCO_cos/1  "<NCO_cos>"
  "Complex Multiplier 6.0 "/2 -> Register1/1
  PA_select/1(Amp) -> [cav2_p1_if_amp]

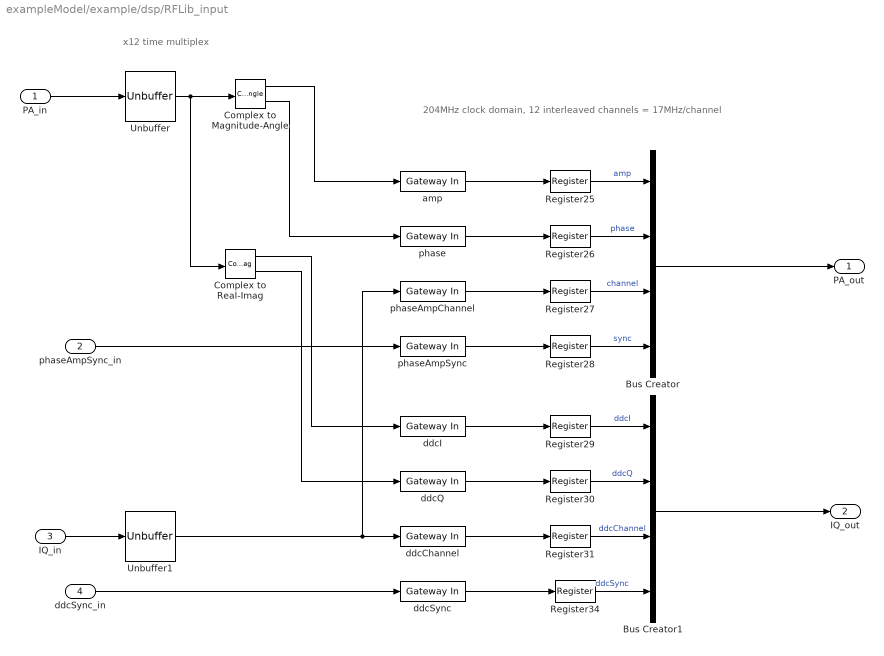
== system exampleModel/example/dsp/RFLib_input ==
  note: x12 time multiplex
  note: 204MHz clock domain, 12 interleaved channels = 17MHz/channel
  PA_in : Inport
  phaseAmpSync_in : Inport  Port=2
  IQ_in : Inport  Port=3
  ddcSync_in : Inport  Port=4
  Bus Creator : BusCreator  Inputs=4
  Bus Creator1 : BusCreator  Inputs=4
  Complex to Magnitude-Angle : ComplexToMagnitudeAngle
  Complex to Real-Imag : ComplexToRealImag
  Register{25..31,34} (8 alike) : xbsIndex_r4/Register  init=0  rst=off  en=off  dbl_ovrd=off  block_type=register
  Unbuffer : Unbuffer
  Unbuffer1 : Unbuffer
  amp : xbsIndex_r4/Gateway In  gui_display_data_type=Fixed-point  arith_type="Signed  (2's comp)"  n_bits=18  bin_pt=17  preci_type=Single  exp_width=8  frac_width=24  rows=1  columns=1  quantization="Round  (unbiased: +/- Inf)"  overflow=Saturate  period=1/Fproc  UseAsADC=off  ADCChannel='1'  interface=None  automatic_assignment=on  address_offset=hex2dec('00')  intf_name=''  intf_description=''  default_value=0  timing_constraint=None  locs_specified=off  LOCs={}  io_standard={}  inherit_from_input=off  hdl_port=on  dbl_ovrd=off  block_type=gatewayin
  ddcChannel : xbsIndex_r4/Gateway In  gui_display_data_type=Fixed-point  arith_type=Unsigned  n_bits=4  bin_pt=0  preci_type=Single  exp_width=8  frac_width=24  rows=1  columns=1  quantization="Round  (unbiased: +/- Inf)"  overflow=Saturate  period=1/Fproc  UseAsADC=off  ADCChannel='1'  interface=None  automatic_assignment=on  address_offset=hex2dec('00')  intf_name=''  intf_description=''  default_value=0  timing_constraint=None  locs_specified=off  LOCs={}  io_standard={}  inherit_from_input=off  hdl_port=on  dbl_ovrd=off  block_type=gatewayin
  ddcI : xbsIndex_r4/Gateway In  gui_display_data_type=Fixed-point  arith_type="Signed  (2's comp)"  n_bits=18  bin_pt=17  preci_type=Single  exp_width=8  frac_width=24  rows=1  columns=1  quantization="Round  (unbiased: +/- Inf)"  overflow=Saturate  period=1/Fproc  UseAsADC=off  ADCChannel='1'  interface=None  automatic_assignment=on  address_offset=hex2dec('00')  intf_name=''  intf_description=''  default_value=0  timing_constraint=None  locs_specified=off  LOCs={}  io_standard={}  inherit_from_input=off  hdl_port=on  dbl_ovrd=off  block_type=gatewayin
  ddcQ : xbsIndex_r4/Gateway In  gui_display_data_type=Fixed-point  arith_type="Signed  (2's comp)"  n_bits=18  bin_pt=17  preci_type=Single  exp_width=8  frac_width=24  rows=1  columns=1  quantization="Round  (unbiased: +/- Inf)"  overflow=Saturate  period=1/Fproc  UseAsADC=off  ADCChannel='1'  interface=None  automatic_assignment=on  address_offset=hex2dec('00')  intf_name=''  intf_description=''  default_value=0  timing_constraint=None  locs_specified=off  LOCs={}  io_standard={}  inherit_from_input=off  hdl_port=on  dbl_ovrd=off  block_type=gatewayin
  ddcSync : xbsIndex_r4/Gateway In  gui_display_data_type=Fixed-point  arith_type=Unsigned  n_bits=1  bin_pt=0  preci_type=Single  exp_width=8  frac_width=24  rows=1  columns=1  quantization="Round  (unbiased: +/- Inf)"  overflow=Saturate  period=1/Fproc  UseAsADC=off  ADCChannel='1'  interface=None  automatic_assignment=on  address_offset=hex2dec('00')  intf_name=''  intf_description=''  default_value=0  timing_constraint=None  locs_specified=off  LOCs={}  io_standard={}  inherit_from_input=off  hdl_port=on  dbl_ovrd=off  block_type=gatewayin
  phase : xbsIndex_r4/Gateway In  gui_display_data_type=Fixed-point  arith_type="Signed  (2's comp)"  n_bits=18  bin_pt=17  preci_type=Single  exp_width=8  frac_width=24  rows=1  columns=1  quantization="Round  (unbiased: +/- Inf)"  overflow=Saturate  period=1/Fproc  UseAsADC=off  ADCChannel='1'  interface=None  automatic_assignment=on  address_offset=hex2dec('00')  intf_name=''  intf_description=''  default_value=0  timing_constraint=None  locs_specified=off  LOCs={}  io_standard={}  inherit_from_input=off  hdl_port=on  dbl_ovrd=off  block_type=gatewayin
  phaseAmpChannel : xbsIndex_r4/Gateway In  gui_display_data_type=Fixed-point  arith_type=Unsigned  n_bits=4  bin_pt=0  preci_type=Single  exp_width=8  frac_width=24  rows=1  columns=1  quantization="Round  (unbiased: +/- Inf)"  overflow=Saturate  period=1/Fproc  UseAsADC=off  ADCChannel='1'  interface=None  automatic_assignment=on  address_offset=hex2dec('00')  intf_name=''  intf_description=''  default_value=0  timing_constraint=None  locs_specified=off  LOCs={}  io_standard={}  inherit_from_input=off  hdl_port=on  dbl_ovrd=off  block_type=gatewayin
  phaseAmpSync : xbsIndex_r4/Gateway In  gui_display_data_type=Fixed-point  arith_type=Unsigned  n_bits=1  bin_pt=0  preci_type=Single  exp_width=8  frac_width=24  rows=1  columns=1  quantization="Round  (unbiased: +/- Inf)"  overflow=Saturate  period=1/Fproc  UseAsADC=off  ADCChannel='1'  interface=None  automatic_assignment=on  address_offset=hex2dec('00')  intf_name=''  intf_description=''  default_value=0  timing_constraint=None  locs_specified=off  LOCs={}  io_standard={}  inherit_from_input=off  hdl_port=on  dbl_ovrd=off  block_type=gatewayin
  PA_out : Outport
  IQ_out : Outport  Port=2
  wires:
  phaseAmpSync_in/1 -> phaseAmpSync/1
  amp/1 -> Register25/1
  phase/1 -> Register26/1
  phaseAmpChannel/1 -> Register27/1
  phaseAmpSync/1 -> Register28/1
  ddcI/1 -> Register29/1
  ddcQ/1 -> Register30/1
  ddcChannel/1 -> Register31/1
  PA_in/1 -> Unbuffer/1
  ddcSync/1 -> Register34/1
  Register25/1 -> Bus Creator/1  "amp"
  Register26/1 -> Bus Creator/2  "phase"
  Register27/1 -> Bus Creator/3  "channel"
  Register28/1 -> Bus Creator/4  "sync"
  Register29/1 -> Bus Creator1/1  "ddcI"
  Register30/1 -> Bus Creator1/2  "ddcQ"
  Register31/1 -> Bus Creator1/3  "ddcChannel"
  Register34/1 -> Bus Creator1/4  "ddcSync"
  IQ_in/1 -> Unbuffer1/1
  Unbuffer1/1 -> phaseAmpChannel/1, ddcChannel/1
  Bus Creator/1 -> PA_out/1
  Unbuffer/1 -> Complex to Real-Imag/1, Complex to Magnitude-Angle/1
  Complex to Magnitude-Angle/1 -> amp/1
  Complex to Magnitude-Angle/2 -> phase/1
  Complex to Real-Imag/1 -> ddcI/1
  Complex to Real-Imag/2 -> ddcQ/1
  Bus Creator1/1 -> IQ_out/1
  ddcSync_in/1 -> ddcSync/1

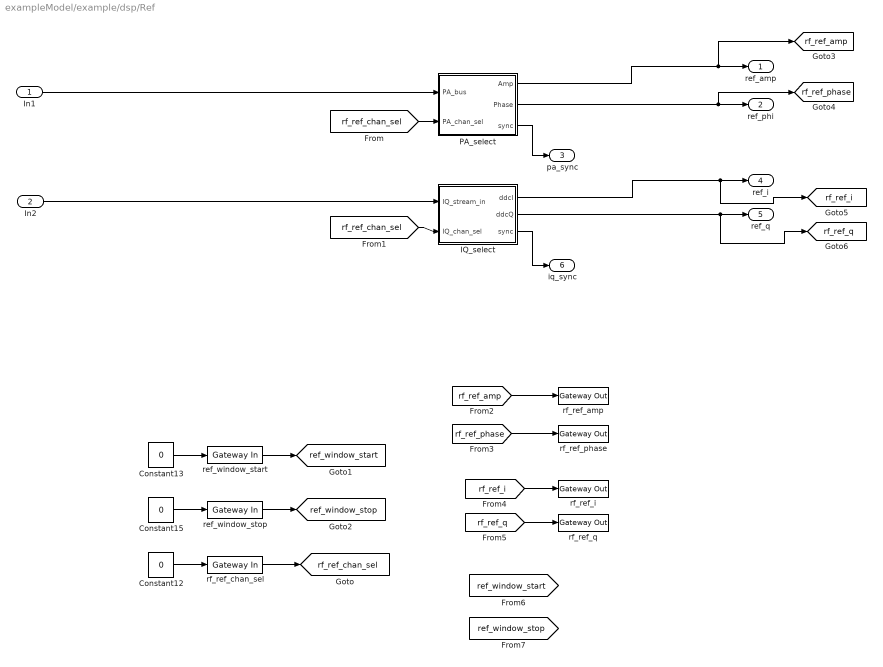
== system exampleModel/example/dsp/Ref ==
  In1 : Inport
  In2 : Inport  Port=2
  Constant12 : Constant  Value=0
  Constant13 : Constant  Value=0
  Constant15 : Constant  Value=0
  IQ_select : Subsystem
  PA_select : Subsystem
  ref_window_start : xbsIndex_r4/Gateway In  gui_display_data_type=Fixed-point  arith_type=Unsigned  n_bits=16  bin_pt=0  preci_type=Single  exp_width=8  frac_width=24  rows=1  columns=1  quantization="Round  (unbiased: +/- Inf)"  overflow=Saturate  period=1/Fproc  UseAsADC=off  ADCChannel='1'  interface=AXI4-Lite  automatic_assignment=off  address_offset=hex2dec('14')  intf_name='ref_window_start'  intf_description=''  default_value=0  timing_constraint=None  locs_specified=off  LOCs={}  io_standard={}  inherit_from_input=off  hdl_port=on  dbl_ovrd=off  block_type=gatewayin
  ref_window_stop : xbsIndex_r4/Gateway In  gui_display_data_type=Fixed-point  arith_type=Unsigned  n_bits=16  bin_pt=0  preci_type=Single  exp_width=8  frac_width=24  rows=1  columns=1  quantization="Round  (unbiased: +/- Inf)"  overflow=Saturate  period=1/Fproc  UseAsADC=off  ADCChannel='1'  interface=AXI4-Lite  automatic_assignment=off  address_offset=hex2dec('18')  intf_name='ref_window_stop'  intf_description=''  default_value=0  timing_constraint=None  locs_specified=off  LOCs={}  io_standard={}  inherit_from_input=off  hdl_port=on  dbl_ovrd=off  block_type=gatewayin
  rf_ref_amp : xbsIndex_r4/Gateway Out  inherit_from_input=off  hdl_port=on  rows=1  columns=1  UseAsDAC=off  DACChannel='1'  interface=AXI4-Lite  automatic_assignment=off  address_offset=hex2dec('00')  intf_name='rf_ref_amp'  intf_description=''  timing_constraint=None  locs_specified=off  LOCs={}  io_standard={}  block_type=gatewayout
  rf_ref_chan_sel : xbsIndex_r4/Gateway In  gui_display_data_type=Fixed-point  arith_type=Unsigned  n_bits=4  bin_pt=0  preci_type=Single  exp_width=8  frac_width=24  rows=1  columns=1  quantization="Round  (unbiased: +/- Inf)"  overflow=Saturate  period=1/Fproc  UseAsADC=off  ADCChannel='1'  interface=AXI4-Lite  automatic_assignment=off  address_offset=hex2dec('10')  intf_name='rf_ref_chan_sel'  intf_description=''  default_value=0  timing_constraint=None  locs_specified=off  LOCs={}  io_standard={}  inherit_from_input=off  hdl_port=on  dbl_ovrd=off  block_type=gatewayin
  rf_ref_i : xbsIndex_r4/Gateway Out  inherit_from_input=off  hdl_port=on  rows=1  columns=1  UseAsDAC=off  DACChannel='1'  interface=AXI4-Lite  automatic_assignment=off  address_offset=hex2dec('08')  intf_name='rf_ref_i'  intf_description=''  timing_constraint=None  locs_specified=off  LOCs={}  io_standard={}  block_type=gatewayout
  rf_ref_phase : xbsIndex_r4/Gateway Out  inherit_from_input=off  hdl_port=on  rows=1  columns=1  UseAsDAC=off  DACChannel='1'  interface=AXI4-Lite  automatic_assignment=off  address_offset=hex2dec('04')  intf_name='rf_ref_phase'  intf_description=''  timing_constraint=None  locs_specified=off  LOCs={}  io_standard={}  block_type=gatewayout
  rf_ref_q : xbsIndex_r4/Gateway Out  inherit_from_input=off  hdl_port=on  rows=1  columns=1  UseAsDAC=off  DACChannel='1'  interface=AXI4-Lite  automatic_assignment=off  address_offset=hex2dec('0C')  intf_name='rf_ref_q'  intf_description=''  timing_constraint=None  locs_specified=off  LOCs={}  io_standard={}  block_type=gatewayout
  ref_amp : Outport
  ref_phi : Outport  Port=2
  pa_sync : Outport  Port=3
  ref_i : Outport  Port=4
  ref_q : Outport  Port=5
  iq_sync : Outport  Port=6
  tag scope: ref_window_start=global, ref_window_stop=global, rf_ref_amp=global, rf_ref_chan_sel=global, rf_ref_i=global, rf_ref_phase=global, rf_ref_q=global
  wires:
  ref_window_stop/1 -> [ref_window_stop]
  In1/1 -> PA_select/1(PA_bus)
  Constant13/1 -> ref_window_start/1
  ref_window_start/1 -> [ref_window_start]
  In2/1 -> IQ_select/1(IQ_stream_in)
  IQ_select/3(sync) -> iq_sync/1
  Constant15/1 -> ref_window_stop/1
  PA_select/3(sync) -> pa_sync/1
  PA_select/1(Amp) -> [rf_ref_amp], ref_amp/1
  PA_select/2(Phase) -> [rf_ref_phase], ref_phi/1
  IQ_select/1(ddcI) -> [rf_ref_i], ref_i/1
  IQ_select/2(ddcQ) -> [rf_ref_q], ref_q/1
  rf_ref_chan_sel/1 -> [rf_ref_chan_sel]
  [rf_ref_chan_sel] -> PA_select/2(PA_chan_sel)
  [rf_ref_chan_sel] -> IQ_select/2(IQ_chan_sel)
  [rf_ref_amp] -> rf_ref_amp/1
  [rf_ref_phase] -> rf_ref_phase/1
  [rf_ref_q] -> rf_ref_q/1
  [rf_ref_i] -> rf_ref_i/1
  Constant12/1 -> rf_ref_chan_sel/1

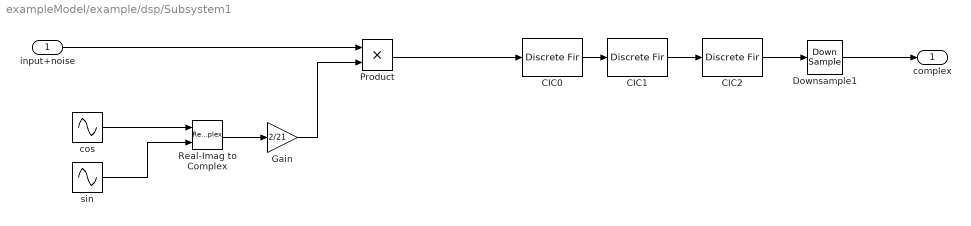
== system exampleModel/example/dsp/Subsystem1 ==
  input+noise : Inport
  CIC0 : DiscreteFir  Coefficients=ones(1,21)/21
  CIC1 : DiscreteFir  Coefficients=ones(1,21)/21
  CIC2 : DiscreteFir  Coefficients=ones(1,21)/21
  Downsample1 : DownSample  N=21  RateOptions=Allow multirate processing
  Gain : Gain  Gain=2/21
  Product : Product
  Real-Imag to Complex : RealImagToComplex
  cos : Sin  Frequency=2*pi*85e6  Phase=-pi/2  SampleTime=Tadc
  sin : Sin  Frequency=2*pi*85e6  SampleTime=Tadc
  complex : Outport
  wires:
  input+noise/1 -> Product/1
  Real-Imag to Complex/1 -> Gain/1
  cos/1 -> Real-Imag to Complex/1
  Gain/1 -> Product/2
  Product/1 -> CIC0/1
  sin/1 -> Real-Imag to Complex/2
  Downsample1/1 -> complex/1
  CIC2/1 -> Downsample1/1
  CIC0/1 -> CIC1/1
  CIC1/1 -> CIC2/1

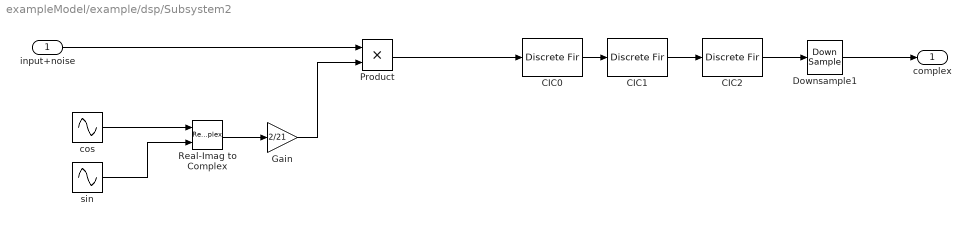
== system exampleModel/example/dsp/Subsystem2 ==
  input+noise : Inport
  CIC0 : DiscreteFir  Coefficients=ones(1,21)/21
  CIC1 : DiscreteFir  Coefficients=ones(1,21)/21
  CIC2 : DiscreteFir  Coefficients=ones(1,21)/21
  Downsample1 : DownSample  N=21  RateOptions=Allow multirate processing
  Gain : Gain  Gain=2/21
  Product : Product
  Real-Imag to Complex : RealImagToComplex
  cos : Sin  Frequency=2*pi*85e6  Phase=-pi/2  SampleTime=Tadc
  sin : Sin  Frequency=2*pi*85e6  SampleTime=Tadc
  complex : Outport
  wires:
  CIC1/1 -> CIC2/1
  CIC0/1 -> CIC1/1
  CIC2/1 -> Downsample1/1
  Downsample1/1 -> complex/1
  sin/1 -> Real-Imag to Complex/2
  Product/1 -> CIC0/1
  Gain/1 -> Product/2
  cos/1 -> Real-Imag to Complex/1
  Real-Imag to Complex/1 -> Gain/1
  input+noise/1 -> Product/1
